simulink model "building_model"  (R2021a)
settings: Solver=FixedStepAuto  StartTime=0.0  StopTime=10  FixedStep=0.018  RelTol=1e-3
undefined symbols (not defined in the file): k1, k2, m1, m2
settings Model: Creator=hdugm  LastModifiedBy=hdugm

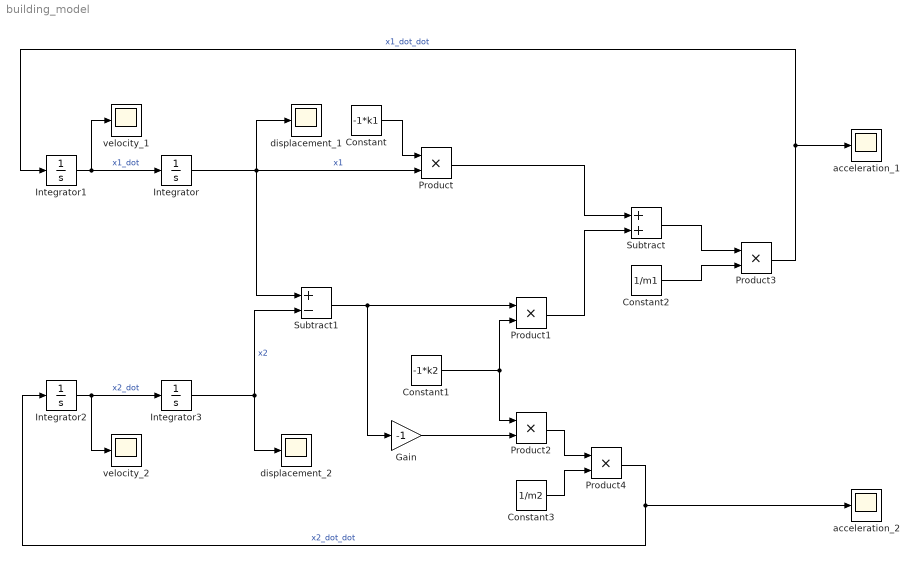
== system building_model ==
  Constant : Constant  Value=-1*k1
  Constant1 : Constant  Value=-1*k2
  Constant2 : Constant  Value=1/m1
  Constant3 : Constant  Value=1/m2
  Gain : Gain  Gain=-1
  Integrator : Integrator  InitialCondition=100
  Integrator1 : Integrator
  Integrator2 : Integrator
  Integrator3 : Integrator  InitialCondition=50
  Product{,1..4} (5 alike) : Product
  Subtract : Sum
  Subtract1 : Sum  Inputs=+-
  acceleration_1 : Scope
  acceleration_2 : Scope
  displacement_1 : Scope
  displacement_2 : Scope
  velocity_1 : Scope
  velocity_2 : Scope
  wires:
  Integrator1/1 -> Integrator/1, velocity_1/1  "x1_dot"
  Integrator/1 -> Subtract1/1, Product/2, displacement_1/1  "x1"
  Constant/1 -> Product/1
  Product/1 -> Subtract/1
  Subtract1/1 -> Product1/1, Gain/1
  Product1/1 -> Subtract/2
  Integrator2/1 -> Integrator3/1, velocity_2/1  "x2_dot"
  Integrator3/1 -> displacement_2/1, Subtract1/2  "x2"
  Constant1/1 -> Product2/1, Product1/2
  Gain/1 -> Product2/2
  Subtract/1 -> Product3/1
  Constant2/1 -> Product3/2
  Product3/1 -> Integrator1/1, acceleration_1/1  "x1_dot_dot"
  Product2/1 -> Product4/1
  Constant3/1 -> Product4/2
  Product4/1 -> Integrator2/1, acceleration_2/1  "x2_dot_dot"
